simulink model "SolarThermTest"  (R2018b)
settings: Solver=FixedStepAuto  StartTime=0.0  StopTime=6.5*3600  FixedStep=5  RelTol=1e-3
undefined symbols (not defined in the file or in its folder): DiscIntNeverNeededParam, path_carnot
libraries: carnot x1
settings Model: Creator=cpp14rcj  LastModifiedBy=cpp14rcj

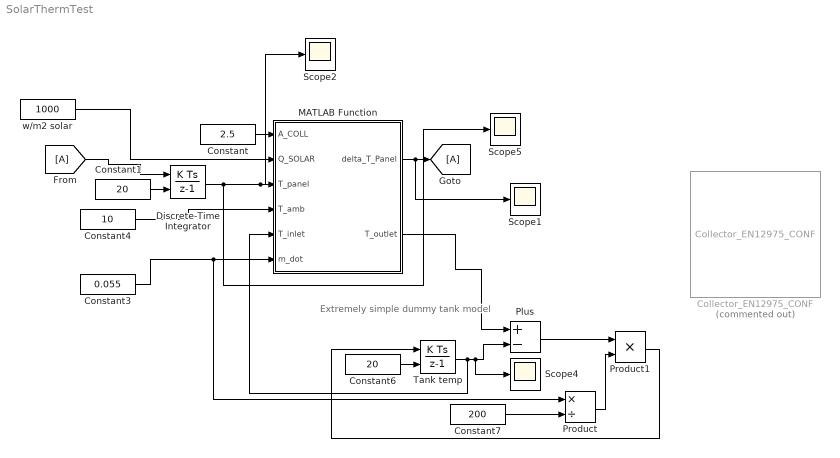
== system SolarThermTest ==
  note: Extremely simple dummy tank model
  Collector_EN12975_CONF : carnot/Source/Solar_Thermal/Collector_EN12975_CONF  Commented=on  tini=20  Ncollector=Ncollector  PathName=fullfile(path_carnot('libsl'), 'Source','Solar_Thermal','Collector_EN12975_CONF','parameter_set')  FileName='DefaultCollector.mat'  userPath=off  userParam=off  acol=3.5  len=0.1  fta=0.7  c1=0.7  c2=0.001  c3=0  c4=0  c5=7000  c6=0  KbAngles=[0 5 10 15 20 25 30 35 40 45 50 55 60 65 70 75 80 85 90]  KbL=[1 1 0.9999 0.9996 0.9991 0.9982 0.9965 0.9935 0.9886 0.9807 0.9678 0.9473 0.9148 0.8638 0.7846 0.6644 0.4907 0.2599 0]  KbT=[1 1 1 1 1 1 1 1 1 1 1 0.875 0.75 0.625 0.5 0.375 0.25 0.125 0]  Kd=0.92  dplin=10  dpqua=10  SensorTimeConstant=10
  Constant : Constant  Value=2.5
  Constant1 : Constant  Value=20
  Constant3 : Constant  Value=0.055
  Constant4 : Constant  Value=10
  Constant6 : Constant  Value=20
  Constant7 : Constant  Value=200
  Discrete-Time Integrator : DiscreteIntegrator  InitialConditionSource=external  InitialCondition=20  SampleTime=-1  ICPrevOutput=DiscIntNeverNeededParam  ICPrevScaledInput=DiscIntNeverNeededParam
  MATLAB Function : MATLAB Function  TreatAsAtomicUnit=on
  Plus : Sum  Inputs=+-
  Product : Product  Inputs=*/
  Product1 : Product  Inputs=**
  Scope{1..2,4..5} (4 alike) : Scope
  Tank temp : DiscreteIntegrator  InitialConditionSource=external  InitialCondition=20  SampleTime=-1  ICPrevOutput=DiscIntNeverNeededParam  ICPrevScaledInput=DiscIntNeverNeededParam
  w/m2 solar : Constant  Value=1000
  wires:
  Constant/1 -> MATLAB Function/1(A_COLL)
  Constant1/1 -> Discrete-Time Integrator/2
  Tank temp/1 -> MATLAB Function/5(T_inlet), Scope4/1, Plus/2
  Constant3/1 -> Product/1, MATLAB Function/6(m_dot)
  Constant4/1 -> MATLAB Function/4(T_amb)
  MATLAB Function/1(delta_T_Panel) -> Scope1/1, [A]
  [A] -> Discrete-Time Integrator/1
  w/m2 solar/1 -> MATLAB Function/2(Q_SOLAR)
  MATLAB Function/2(T_outlet) -> Plus/1
  Discrete-Time Integrator/1 -> Scope5/1, Scope2/1, MATLAB Function/3(T_panel)
  Constant6/1 -> Tank temp/2
  Constant7/1 -> Product/2
  Plus/1 -> Product1/1
  Product/1 -> Product1/2
  Product1/1 -> Tank temp/1

== matlab function SolarThermTest/MATLAB Function ==
  data: A_COLL input; delta_T_Panel output; Q_SOLAR input; T_panel input; T_amb input; T_inlet input; m_dot input; T_outlet output
function [delta_T_Panel,T_outlet]  = fcn(A_COLL,Q_SOLAR,T_panel,T_amb,T_inlet,m_dot)



c=[3.5*A_COLL
    0.02*A_COLL
    0
    0
    7000
    0];

optical_efficiency=0.8;

    T_diff = (T_panel - T_amb); % difference between mean collector temperature and ambient */
	POWER = 2.0*m_dot*4180*(T_panel - T_inlet); %this is the heat lost from the panel energy due to flow of water in and out of the panel, the 2 arises due to transforming (Tout-Tin) to (2Tm-2Tin) using Tout=2Tm-Tin

    
    delta_T_Panel = ((Q_SOLAR*A_COLL)*optical_efficiency - T_diff *(c(1,1) + c(2,1)*T_diff)-POWER) / (c(5,1)*A_COLL);
    T_outlet=2*T_panel-T_inlet;
